simulink model "GuytonModel1972WithSubsystems_R2018_new"  (Simulink 9.1)
settings: Solver=ode23tb  StartTime=0.0  StopTime=inf  RelTol=1e-3  EnableMultiTasking=on
(part 1 of 3)
settings Model: LogicAnalyzerSignalOrdering=7aa3712b-a82d-49b1-ab79-c4b2009123cc,5a57f72a-0b0f-46f2-acdb-43125fd8ce03,a1eed3b7-a639-4f6e-9e66-41bbe214b6e5,0125497b-a83f-4e6f-858a-d937ae2b0d76,3e99b8dd-3e9c-45af-bc6c-72cad900a970,bdf28fdf-f6ee-494c-b426-144877683f61,daad667d-899e-428c-8c0c-82b3f4a58e16,7a1ec332-910d-4d5f-b535-061f2b58242f,8797777e-8256-4824-9350-18babea3f7fb,fa05effb-f5f0-4fb9-ae93-2c2ec5624b9e,8be5053f-f699-4e3b-912d-bda2fdf05311,7071d1a3-cbf6-4004-9a33-fb4c74e307a2,12eca2b8-30c7-4ca1-80c7-0d748863521c,1491594a-a680-41cf-9df3-666274efcfc0,a408ffc1-1556-4b3f-a007-6827623c9fa9,7caa9f0e-c1ef-45aa-8dd4-854c340c4311,cf932523-36ef-4960-9416-a49f3ce3abf4,5572dfed-c94c-4ac7-aa9a-9887f7f6c75f,825e1703-83b2-4867-8ebe-c975c17187a2,5d5b3bbb-1bff-46a6-a854-092626d3bdcf,2f97d808-bd79-4a93-951d-b9bb7f21fa84,3d0caab8-259e-423e-95e2-69965d32bdad,c121611d-42a5-4154-afc6-d4da5485fa77,4f2143c4-e6aa-439a-b86a-19df9d8919b1,a38d8fc3-90f2-40d7-afcb-4fa07d609ab0,d1aaf1a0-ab7d-4766-b05b-b674d56eddeb,9154d59b-3667-486d-a870-b223c724f572,4947b9e5-a051-4927-826b-f88022b127af,a5c37f39-2afb-4bf5-b5f4-deaa4e4f9e26,ab2d206b-5aa5-47ca-82a6-285e3435147c,a24f4fe4-8f8f-4ad5-bc1c-63b53242714e,d663d5fd-813e-4f3b-aebe-eaf2e7a06971,ca1ad65c-e5ef-44d1-86e8-ee4ec15310cd,a373b868-86f5-4960-8c53-9f982b71114b,b32a667a-ee1b-4402-8ab6-0e0293fa6f38,7e1f8eb4-0f51-4604-b00f-97ee570519ec,69dfedaa-aa11-44aa-8eef-81c2d931c5df,4045ec49-f8a0-442b-8ade-123442e10924,2a26ec00-979f-4a7b-8e9c-28a5bec13211,7373e241-3f2f-4e4f-91f7-b5466dda58a8,c9a36257-ac58-4413-a313-935ac06f1bc8  Creator=Jirka  LastModifiedBy=Jirka
settings DataIOCC: LimitDataPoints=on  MaxDataPoints=1000000  SaveFormat=Structure
settings OptimizationCC: ExpressionDepthLimit=2147483647  InitFltsAndDblsToZero=on
settings DebuggingCC: SaveWithParameterizedLinksMsg=none  SignalResolutionControl=TryResolveAllWithWarning  SolverPrmCheckMsg=warning  MultiTaskDSMMsg=warning  MultiTaskCondExecSysMsg=none  FcnCallInpInsideContextMsg=warning  StateNameClashWarn=warning
settings GRTTargetCC: TargetFcnLib=ansi_tfl_tmw.mat

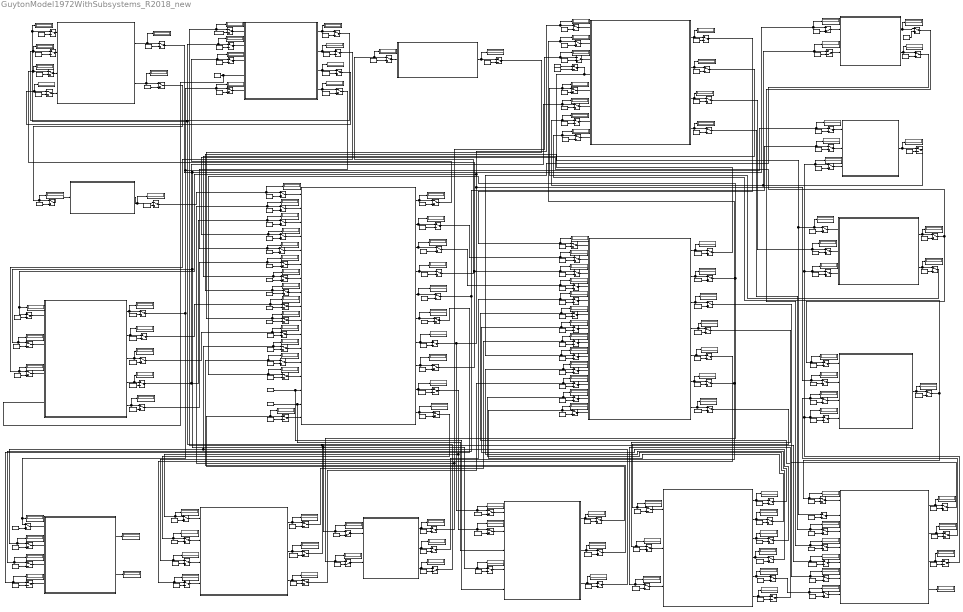
== system GuytonModel1972WithSubsystems_R2018_new ==
  note: PVS
  note: RVS
  note: BFN
  note: BFM
  note: PA
  note: PPA
  note: PRA
  note: PLA
  note: QLO
  note: VVE
  note: PC
  note: VV7
  note: VB
  note: VVR
  note: RBF
  note: AVE
  note: HPR
  note: HMD
  note: HPL
  note: ANM
  note: AMM
  note: AUM
  note: ARM
  note: VIM
  note: AUH
  note: HSR
  note: HSL
  note: AMM
  note: AOM
  note: P2O
  note: OVA
  note: AU
  note: EXC
  note: BFM
  note: HM
  note: VPF
  note: AUM
  note: PPC
  note: AM
  note: CNE
  note: AHM
  note: VIM
  note: REK
  note: PA
  note: AHM
  note: POT
  note: TVD
  note: STH
  note: AU
  note: CNA
  note: PRA
  note: RFN
  note: REK
  note: CNA
  note: CNE
  note: ANM
  note: RVS
  note: VUD
  note: BFN
  note: PVS
  note: VRC
  note: PIF
  note: PTC
  note: DFP
  note: TVD
  note: VTL
  note: PPD
  note: CPI
  note: DPL
  note: VB
  note: DPC
  note: PC
  note: VP
  note: CPP
  note: PPC
  note: VTC
  note: ANM
  note: PA
  note: CKE
  note: CNA
  note: AM
  note: DPC
  note: VTC
  note: VID
  note: CPI
  note: PTC
  note: DPL
  note: VTL
  note: VTS
  note: PIF
  note: PA
  note: PPA
  note: POT
  note: HPR
  note: HPL
  note: HMD
  note: POT
  note: VB
  note: HM
  note: VIM
  note: VRC
  note: PPA
  note: PLA
  note: CPP
  note: PPC
  note: VPF
  note: PPD
  note: DFP
  note: QLO
  note: HMD
  note: AU
  note: PRA
  note: AUM
  note: AVE
  note: AUH
  note: VVR
  note: AU
  note: POT
  note: EXC
  note: P2O
  note: PA
  note: POV
  note: ARM
  note: VID
  note: NOD
  note: STH
  note: VPF
  note: VP
  note: VTS
  note: CNA
  note: CKE
  note: VTW
  note: AM
  note: REK
  note: VUD
  note: RBF
  note: RFN
  note: NOD
  note: AHM
  note: NON-MUSCLE OXYGEN DELIVERY
  note: MUSCLE BLOOD FLOW CONTROL AND PO2
  note: VASCULAR STRESS RELAXATION
  note: KIDNEY DYNAMICS AND EXCRETION
  note: THIRST AND DRINKING
  note: ANTIDIURECTIC HORMONE CONTROL
  note: ALDOSTERONE CONTROL
  note: ANGIOTENSIN CONTROL
  note: ELECTROLYTES AND CELL WATER
  note: TISSUE FLUIDS, PRESSURES AND GEL
  note: HEART HYPERTROPHY OR DETERIORATION
  note: RED CELLS AND VISCOSITY
  note: PULMONARY DYNAMICS AND FLUIDS
  note: HEART RATE AND STROKE VOLUME
  note: AUTONOMIC CONTROL
  note: NON-MUSCLE LOCAL
      | BLOOD FLOW CONTROL
  note: CIRCULATORY DYNAMICS
  note: CAPILLARY MEMBRANE DYNAMICS
  AOM : Constant
  Aldosterone Control : Subsystem
      settings: MinAlgLoopOccurrences=on
      mask Display: disp('ALDOSTERONE CONTROL\n\nINTPUT:\nANM - angiotensin multiplier effect on vascular resistance,\n ratio to normal\nPA - aortic pressure [torr]\nCKE - extracellural potassium concentration \nCNA - extracellural sodium concentration \n\nOUTPUT:\nAM - aldosterone multiplier, ratio of normal effect\n')
  Angiotensin Control : Subsystem
      settings: MinAlgLoopOccurrences=on
      mask Display: disp('ANGIOTENSIN CONTROL\n\nINTPUTS:\nREK - percent of normal renal function\n [ratio to normal] \nRFN - renal blood flow if kidney is not damaged [l/min]\nCNA - extracellural sodium concentration \n\n\n OUTPUTS:\nANM - angiotensin multilier factor on vascular resistance\n [ratio to normal]\nCNE - sodium concentration abnormality causing third factor effect\n')
  Antidiurectic Hormone Control : Subsystem
      settings: MinAlgLoopOccurrences=on
      mask Display: disp('ANTIDIURECTIC HORMONE CONTROL\n\nINTPUT:\nAU - overall activity of autonomic system,\n ratio to normal \nPRA - right artial pressure \nCNA - extracellural sodium contrentration \n\nOUTPUT:\nAHM - antidiurectic hormone multiplifier,\n ratio of normal effect\n')
  Autonomic Control : Subsystem
      mask Display: disp('AUTONOMIC CONTROL \n\nINTPUTS:\nPA - systemic arterial pressure torr\nPOT - non-muscle cell PO2 [torr]\nP2O - muscle cell PO2  [torr]\nEXC - Effect of excercise on the metabolic usage of oxygen \nby the muscles [ratio to resting state]\nAUZ - overall sensitivity of autonomic control [ratio to normal]\n\nOUTPUTs:\nAU - overall activity af autonomic system\n[ratio to normal]\nAUH - autonomic multilier effect on the heart output\n[ratio to normal]\nVVR - basic volume of venous tree(maximum volume\n at zero pressure) [l]\nAUM - autonomic multipllier effect on arterial resistance \n[ratio to normal]\nAVE - autonomic multipllier effect on venous resistance\n[ratio to normal]\n')
  BFN : Constant  Value=2.8
  Capillary Membrane Dynamics : Subsystem
      mask Display: disp('CAPILLARY MEMBRANE DYNAMICS\n\nINTPUTS:\nPTC - colloid osmotic pressure of the tissue gel [torr]\nVTL - rate of return of fluid from the interstitium to the\nblood through the lymph [l/min]\nTVD - rate of intake of fluid by mounth or otherwise [l/min]\nRVS - venous resistance\nBFN - blood flow in non-muscle, non renal tissues\nPVS - average venous pressure\nVRC - volume of red blood cell\nVUD - rate of urinary output\nDFP - rate of increase in pulmonary free field\nPIF - intersticial fluid pressure\nPPD - rate od change of protein in pulmonary fluids\nCPI - concentration of protein in free intersticial fluid\nVP - plasma volume [l]\nDPL - rate of systemic lymphatic return of protela\n\nOUTPUTS:\nPC - systemic capillary pressure [torr]\nPPC - plasma colloid osmotic pressure [torr] \nVTC - toral rate of movement of fluid out of systemic capillaries[l/min]\nVB - blood volume\nCPP - plasma protein concentration\nDPC - rate of loss of plasma protein through systemic capillaries\n')
  Circulatory Dynamics : Subsystem
      settings: MinAlgLoopOccurrences=on
      mask Display: disp('CIRCULATORY DYNAMICS\n\nINTPUTS:\nARM - vasoconstrictor effect of all types of autoregulation\nVIM - blood viscosity (ratio to normal blood)\nAUM - sympathetic vasoconstrictor effect on arteries\nANM - angiotensin multiplier effect on vascular resistance, ratio to normal\nAMM - muscle vascular constriction caused by local tissue control, ratio to resting state\nAVE - sympathetic vasoconstrictor effect on veins\nRBF - renal blood flow [l/min]\nPC - capillary pressure  [torr]\nVVR - diminished vascular volume caused by sympathetic stimulation [l]\nVV7 - increased vascular volume caused by stress relaxation [l]\nAUH - autonomic stimulation of heart, ratio to normal\nHMD - cardiac depresant effect of hypoxia\nHPL - hypertrophy effect on left ventricle [ratio to normal]\nHPL - hypertrophy effect of left heart [ratio to normal]\nVB - blood volume [l]\nHSR - basic strenght or right ventricle [ratio to normal]\nHPR - hypertrophy effect of right heart [ratio to normal]\n\n\n  OUTPUTS:\nBFM - muscle blood flow [l/min]\nRVS - venous resistance [torr/l/min]\nPVS - average venous pressure  [torr]\nVVE - excess blood (stressed) volume in the systemic veins [l] \nPRA - right atrial pressure  [torr]\nQLO - output of left ventricle [l/min]\nPA - aortic pressure  [torr] \nBFN - blood flow in non-muscle, non-renal tissues [l/min]\nPRA - right atrial pressure  [torr]\nPLA - left atrial pressure  [torr]\n')
  Constant{1..2,4,95,106,189..190,196,198..201,205,209,213,216,234..235,241,245..249,254..257,259..260,274,280,283,285,295..297,299,304..306,308..309,322} (44 alike) : Constant
  Constant187 : Constant  Value=0.0125
  Constant188 : Constant  Value=40
  Constant192 : Constant  Value=0.3
  Constant{193,210,223,238,323} (5 alike) : Constant  Value=100
  Constant194 : Constant  Value=28
  Constant197 : Constant  Value=10
  Constant{202,221,231,236,253,268,271,275,281,286,302..303,320,325} (14 alike) : Constant  Value=0
  Constant{203,207,212,288} (4 alike) : Constant  Value=142
  Constant{204,226..227,239..240} (5 alike) : Constant  Value=8
  Constant{208,250,278..279} (4 alike) : Constant  Value=1.2
  Constant{211,229,237,258,267,287,290,315,324} (9 alike) : Constant  Value=5
  Constant215 : Constant  Value=0.1
  Constant217 : Constant  Value=0.0125
  Constant218 : Constant  Value=3
  Constant219 : Constant  Value=12
  Constant{220,270,291,313} (4 alike) : Constant  Value=0.002
  Constant{222,273,292,312} (4 alike) : Constant  Value=0.04
  Constant224 : Constant  Value=15
  Constant225 : Constant  Value=200
  Constant228 : Constant  Value=7.979
  Constant230 : Constant  Value=15
  Constant232 : Constant  Value=28
  Constant233 : Constant  Value=70
  Constant243 : Constant  Value=40
  Constant244 : Constant  Value=1.6
  Constant251 : Constant  Value=17
  Constant252 : Constant  Value=2.95
  Constant261 : Constant  Value=0.001
  Constant262 : Constant  Value=2.9
  Constant263 : Constant  Value=2.8
  Constant264 : Constant  Value=3.7
  Constant265 : Constant  Value=2
  Constant266 : Constant  Value=-6.3
  Constant269 : Constant  Value=0.001
  Constant272 : Constant  Value=20
  Constant276 : Constant  Value=0.001
  Constant277 : Constant  Value=0.1
  Constant284 : Constant  Value=10
  Constant289 : Constant  Value=12
  Constant293 : Constant  Value=-6.3
  Constant294 : Constant  Value=20
  Constant298 : Constant  Value=2
  Constant3 : Constant  Value=0.3
  Constant300 : Constant  Value=40
  Constant301 : Constant  Value=0.0125
  Constant307 : Constant  Value=2.95
  Constant310 : Constant  Value=3
  Constant311 : Constant  Value=70
  Constant314 : Constant  Value=17
  Constant316 : Constant  Value=28
  Constant317 : Constant  Value=3.7
  Constant318 : Constant  Value=2.9
  Constant319 : Constant  Value=0.3
  Constant321 : Constant  Value=2.8
  Constant326 : Constant  Value=15
  Display{1..143} (143 alike) : Display
  Electrolytes and Cell Water : Subsystem
      settings: MinAlgLoopOccurrences=on
      mask Display: disp('ELECTROLYTES AND CELL WATER\n\nINTPUTS:\nAM - aldosterone multiplier, ratio of normal effect\nREK - percent of normal renal function\n [ratio to normal] \nNOD - rate of excretion of sodium in the urine [mmol/min]\nSTH - salt appetite multiplier factor [ratio to normal]\nVTS - systemic interstitial fluid volume [l]\nVP - plasma volume [l]\nVPF - pulmonary interstitial fluid volume [l]\n\nOUTPUTS:\nVID - rate of fluid transfer between interstitial fluid and cells [l/min]\nCKE - extracellular potassium concentration [mmol/l]\nCNA - extracellular sodium concentration [mmol/l]\nVTW - total body water [l]\n')
  HM : Constant  Value=40
  Heart Hypertrophy or Deterioration : Subsystem
      settings: MinAlgLoopOccurrences=on
      mask Display: disp('HEART HYPERTROPHY OR DETERIORATION\n\nINTPUTS:\nPA - systemic arterial pressure [torr]\nPPA - pulmonary arterial pressure [torr]\nHSL - basic strenght or left ventricle [ratio to normal]\nPOT - Non muscle cells PO2 [troo]\nHSR - basic strenght or right ventricle [ratio to normal]\n\nOUTPUTS:\nHPR - hypertrophy effect of right heart [ratio to normal]\nHPL - hypertrophy effect of left heart [ratio to normal]\nHMD - cardiac depresant effect of hypoxia, shock\n')
  Heart Rate and Stroke Volume : Subsystem
      settings: MinAlgLoopOccurrences=on
      mask Display: disp('HEART RATE AND STROKE VOLUME\n\nINTPUTS:\nAUR - overall activity of autonomic system \n[ratio to normal] \nHMD - cardiac depresant effect of hypoxia, shock\nand other factors [ratio to normal] \nPRA - right atrial pressure [torr]\nQLO - output of left ventricle [l/min]\n\nOUTPUTS:\nSVO - stroke volume [l]\nHT - heart rate\n')
  Kidney  Dynamics and Excretion : Subsystem
      settings: MinAlgLoopOccurrences=on
      mask Display: disp('KIDNEY DYNAMICS AND EXCRETION\n\nINTPUTS:\nPA - aortic pressure [torr]\nPPC - plasma colloid osmotic pressure [torr] \nVIM - blood viscosity (ratio to normal blood \n[torr min/ll] \nREK - percent of normal renal function [ratio to normal] \nCNE - sodium concentration abnormability \ncausing third factor effect [mmol/l]\nAUM - sympathetic vasoconstrictor effect \non arteries [ratio of normal effect]\nAHM - antidiuretic hormone [ratio of normal effect]\nAM - aldosterone multiplier [ratio of normal effect] \n\n\n  OUTPUTS:\nVUD - rate of urinary output [l/min]\nRBF- renal blood flow [l/min]\nRFN - renal blood flow if kidney is not damaged [l/min]\nNOD - rate of renal excretion of sodium [mmol/min]\n\nAAR - afferent arteriolar resistance [torr min/l]\nEVR - postglomerular resistance [torr min/l]\nRR - renal resistance [torr min/l]\nGLP - glomerular pressure [torr]\nGFN - glomerular filtration rate of undamaged kidney [l/min]\nGFR - glomerular filtration rate [l/min]\n')
  Manual Switch{1..12,14..20,23..44,47..110,112..138,142..145} (136 alike) : ManualSwitch
  Manual Switch{13,21..22,45..46,111} (6 alike) : ManualSwitch  CurrentSetting=0
  Muscle Blood Flow Control And pO2 : Subsystem
      settings: MinAlgLoopOccurrences=on
      mask Display: disp('MUSCLE BLOOD FLOW CONTROL AND PO2\n\nINTPUTS:\nVPF - volume of free fluid in the pulmonary interstitium \nHM - hematocrit [%]\nBFM - blood flow in muscles \n [l/min]\nEXC - Effect of excercise on the metabolic usage \nof oxygen by the muscles [ratio to resting state]\nAU - overall activity of autonomic system\n  \nOUTPUTS:\nOVA - oxygen content of arterial blood \n[ml O2 STPD/l blood] \nP2O - muscle cell PO2  [torr]\nAOM - autonomic effect on tissue oxygenation \nAMM - muscle vascular constriction caused by logical tissue control\n[multiplifier, ratio to normal]\n\n')
  NON-MUSCLE OXYGEN DELIVERY : Subsystem
      mask Display: disp('NON-MUSCLE OXYGEN DELIVERY\n\nINTPUTS:\nHM-hematocrit [%]\nOVA-oxygen volume in aortic blood [ml O2/l blood]\nBFN-blood flow in non-muscle, non-renal tissues [l/min]\nAOM-autonomic effect on tissue oxygen utilization\n\nOUTPUTS:\nPOT-non-muscle cell PO2  [torr]\nPOV-non-muscle venous PO2 [torr]\n')
  "Non-Muscle Local Blood Flow Control " : Subsystem
      settings: MinAlgLoopOccurrences=on
      mask Display: disp('NON MUSCLE LOCAL BLOOD FLOW CONTROL\n\nINTPUT:\nPOT - non-muscle cells PO2 [torr] \n\nOUTPUT:\nARM - vasoconstrictor effect of local blood flow\n autoregulationin non-muscle tissues \n[ratio to normal]\n')
  OVA : Constant  Value=200
  POT : Constant  Value=8
  POV : Constant  Value=40
  Pulmonary Dynamics and Fluids : Subsystem
      mask Display: disp('PULMONARY DYNAMICS AND FLUIDS\n\nINTPUTS:\nPPA - pulmonary arterial pressure [torr]\nPLA - left atrial pressure [torr]\nPPC - plasma colloid osmotic pressure [torr]\nCPP - plasma protein concentration\n\nOUTPUTs:\nDFP - rate of change of free fluid in the lungs [l/min]\nVPF - volume of free fluid in the pulmonary interstitium [l/min]\nPPD - rate of loss of protein through the pulmonary capillary \nmembrane [g/min]\n')
  Red Cells And Viscosity : Subsystem
      settings: MinAlgLoopOccurrences=on
      mask Display: disp('RED CELLS AND VISCOSITY\n\nINTPUT:\nPOT - non-muscle cell PO2 [torr]\nVB - volume of blood [l]\n\nOUTPUT:\nVIM - blood viscosity [ratio to normal]\nHM - hematocrit [%]\nVRC - volume of red blood cells []\n')
  Thirst And Drinking : Subsystem
      settings: MinAlgLoopOccurrences=on
      mask Display: disp('THIRST AND DRINKING\n\nINTPUT:\nPOT - non muscle cells PO2 [torr] \nAHM - antidiurectical hormone effect to non renal\n vascular resistance, multiplifier \n(ratio to normal effect)\nOUTPUT:\nSTH - salt appetite multiplifier factor\n [ratio to normal]  \nTVD - rate of intake of fluid by mouth \n or otherwise [l/min]\n')
  "Tissue Fluids, Pressures and Gel" : Subsystem
      mask Display: disp('TISSUE FLUIDS, PRESSURES AND GEL\n\nINTPUTS:\nVTC - rate of fluid transfer across systemic intersticial fluid\nDPC -rate of influx protein into the interstitial fluid from plasma [g/min]\nVID - rate of fluid transfer between interstitial fluid and cells\n\nOUTPUTs:\nPTC - total colloid osmotic pressure of the tissue gel]\nVTL - lymph flow rate [l/min]\nDPL - rate of return of protein to the circulatin by way of the lymph [g/min]\nCPI - concentration pf protein in the interstitium [g/l]\nVTS - total interstitial fluid volume [l]\n')
  Vascular Stress Relaxation : Subsystem
      settings: MinAlgLoopOccurrences=on
      mask Display: disp('VASCULAR STRESS RELAXATION\n\nINTPUT:\nVVE - VVE - excess blood (stressed) volume in the veins [l] \n \n\nOUTPUT:\nVV7 - increased vascular volume caused by stress relaxation [l] \n')
  wires:
  Circulatory Dynamics/3(PVS) -> Manual Switch129/1, Display2/1
  Constant317/1 -> Manual Switch129/2
  Circulatory Dynamics/2(RVS) -> Manual Switch130/1, Display1/1
  Constant318/1 -> Manual Switch130/2
  Constant321/1 -> Manual Switch133/2
  Circulatory Dynamics/1(BFM) -> Manual Switch134/1, Display35/1
  Constant322/1 -> Manual Switch134/2
  Circulatory Dynamics/7(PA) -> Manual Switch135/1, Display6/1
  Constant323/1 -> Manual Switch135/2
  Circulatory Dynamics/8(BFN) -> Manual Switch133/1, Display7/1
  Constant326/1 -> Manual Switch138/2
  Circulatory Dynamics/5(PRA) -> Manual Switch132/1, Display4/1
  Constant320/1 -> Manual Switch132/2
  Circulatory Dynamics/9(PPA) -> Manual Switch138/1, Display8/1
  Circulatory Dynamics/10(PLA) -> Manual Switch137/1, Display9/1
  Constant325/1 -> Manual Switch137/2
  Circulatory Dynamics/6(QLO) -> Manual Switch136/1, Display5/1
  Constant324/1 -> Manual Switch136/2
  Circulatory Dynamics/4(VVE) -> Manual Switch131/1, Display3/1
  Constant319/1 -> Manual Switch131/2
  Manual Switch68/1 -> Circulatory Dynamics/8(PC)
  Constant251/1 -> Manual Switch68/2
  Manual Switch70/1 -> Circulatory Dynamics/10(VV7)
  Constant253/1 -> Manual Switch70/2
  Manual Switch75/1 -> Circulatory Dynamics/14(VB)
  Constant258/1 -> Manual Switch75/2
  Manual Switch69/1 -> Circulatory Dynamics/9(VVR)
  Constant252/1 -> Manual Switch69/2
  Manual Switch67/1 -> Circulatory Dynamics/7(RBF)
  Constant250/1 -> Manual Switch67/2
  Manual Switch66/1 -> Circulatory Dynamics/6(AVE)
  Constant249/1 -> Manual Switch66/2
  Manual Switch77/1 -> Circulatory Dynamics/17(HPR)
  Constant260/1 -> Manual Switch77/2
  Manual Switch72/1 -> Circulatory Dynamics/12(HMD)
  Constant255/1 -> Manual Switch72/2
  Manual Switch73/1 -> Circulatory Dynamics/13(HPL)
  Constant256/1 -> Manual Switch73/2
  Manual Switch64/1 -> Circulatory Dynamics/4(ANM)
  Constant247/1 -> Manual Switch64/2
  Manual Switch65/1 -> Circulatory Dynamics/5(AMM)
  Constant248/1 -> Manual Switch65/2
  Manual Switch63/1 -> Circulatory Dynamics/3(AUM)
  Constant246/1 -> Manual Switch63/2
  Manual Switch61/1 -> Circulatory Dynamics/1(ARM)
  Constant244/1 -> Manual Switch61/2
  Manual Switch62/1 -> Circulatory Dynamics/2(VIM)
  Constant245/1 -> Manual Switch62/2
  Manual Switch71/1 -> Circulatory Dynamics/11(AUH)
  Constant254/1 -> Manual Switch71/2
  Constant259/1 -> Circulatory Dynamics/15(HSR), Heart Hypertrophy or Deterioration/5(HSR)
  Constant257/1 -> Circulatory Dynamics/16(HSL), Heart Hypertrophy or Deterioration/3(HSL)
  Manual Switch142/1 -> NON-MUSCLE OXYGEN DELIVERY/1(HM)
  Manual Switch143/1 -> NON-MUSCLE OXYGEN DELIVERY/2(OVA)
  Manual Switch144/1 -> NON-MUSCLE OXYGEN DELIVERY/3(BFN)
  Manual Switch145/1 -> NON-MUSCLE OXYGEN DELIVERY/4(AOM)
  NON-MUSCLE OXYGEN DELIVERY/1(POT) -> Display11/1, Manual Switch1/1
  POT/1 -> Manual Switch1/2
  NON-MUSCLE OXYGEN DELIVERY/2(POV) -> Display10/1, Manual Switch2/1
  POV/1 -> Manual Switch2/2
  HM/1 -> Manual Switch142/2
  OVA/1 -> Manual Switch143/2
  BFN/1 -> Manual Switch144/2
  AOM/1 -> Manual Switch145/2
  Manual Switch4/1 -> Muscle Blood Flow Control And pO2/1(VPF)
  Manual Switch5/1 -> Muscle Blood Flow Control And pO2/2(HM)
  Manual Switch6/1 -> Muscle Blood Flow Control And pO2/3(BFM)
  Manual Switch8/1 -> Muscle Blood Flow Control And pO2/5(AU)
  Muscle Blood Flow Control And pO2/4(AMM) -> Manual Switch42/1, Display19/1
  Constant241/1 -> Manual Switch42/2
  Muscle Blood Flow Control And pO2/3(AOM) -> Manual Switch43/1, Display17/1
  Constant274/1 -> Manual Switch43/2
  Muscle Blood Flow Control And pO2/2(P2O) -> Manual Switch31/1, Display15/1
  Constant226/1 -> Manual Switch31/2
  Constant225/1 -> Manual Switch23/2
  Muscle Blood Flow Control And pO2/1(OVA) -> Manual Switch23/1, Display16/1
  Constant189/1 -> Manual Switch6/2
  Constant188/1 -> Manual Switch5/2
  Constant187/1 -> Manual Switch4/2
  Constant1/1 -> Manual Switch8/2
  Constant192/1 -> Manual Switch9/2
  Manual Switch9/1 -> Vascular Stress Relaxation/1(VVE)
  Vascular Stress Relaxation/1(VV7) -> Manual Switch58/1, Display21/1
  Constant275/1 -> Manual Switch58/2
  Constant198/1 -> Manual Switch15/2
  Manual Switch15/1 -> Kidney  Dynamics and Excretion/6(AUM)
  Manual Switch11/1 -> Kidney  Dynamics and Excretion/2(PPC)
  Constant194/1 -> Manual Switch11/2
  Manual Switch17/1 -> Kidney  Dynamics and Excretion/8(AM)
  Constant200/1 -> Manual Switch17/2
  Manual Switch14/1 -> Kidney  Dynamics and Excretion/5(CNE)
  Constant197/1 -> Manual Switch14/2
  Manual Switch16/1 -> Kidney  Dynamics and Excretion/7(AHM)
  Constant199/1 -> Manual Switch16/2
  Manual Switch13/1 -> Kidney  Dynamics and Excretion/3(VIM)
  Constant196/1 -> Manual Switch13/2
  Manual Switch10/1 -> Kidney  Dynamics and Excretion/1(PA)
  Constant193/1 -> Manual Switch10/2
  Kidney  Dynamics and Excretion/3(RFN) -> Manual Switch74/1, Display30/1
  Constant279/1 -> Manual Switch74/2
  Kidney  Dynamics and Excretion/4(NOD) -> Manual Switch91/1, Display31/1
  Constant277/1 -> Manual Switch91/2
  Kidney  Dynamics and Excretion/1(VUD) -> Manual Switch76/1, Display32/1
  Constant276/1 -> Manual Switch76/2
  Kidney  Dynamics and Excretion/2(RBF) -> Manual Switch59/1, Display23/1
  Constant278/1 -> Manual Switch59/2
  Manual Switch21/1 -> Thirst And Drinking/1(POT)
  Constant204/1 -> Manual Switch21/2
  Manual Switch22/1 -> Thirst And Drinking/2(AHM)
  Thirst And Drinking/2(TVD) -> Manual Switch93/1, Display34/1
  Thirst And Drinking/1(STH) -> Manual Switch92/1, Display37/1
  Constant205/1 -> Manual Switch22/2
  Manual Switch20/1 -> Antidiurectic Hormone Control/3(CNA)
  Constant203/1 -> Manual Switch20/2
  Constant201/1 -> Manual Switch18/2
  Manual Switch18/1 -> Antidiurectic Hormone Control/1(AU)
  Manual Switch19/1 -> Antidiurectic Hormone Control/2(PRA)
  Constant202/1 -> Manual Switch19/2
  Antidiurectic Hormone Control/1(AHM) -> Manual Switch94/1, Display39/1
  Constant2/1 -> Manual Switch94/2
  Manual Switch25/1 -> Angiotensin Control/2(RFN)
  Constant208/1 -> Manual Switch25/2
  Manual Switch24/1 -> Angiotensin Control/3(CNA)
  Constant207/1 -> Manual Switch24/2
  Angiotensin Control/2(CNE) -> Manual Switch96/1, Display43/1
  Constant284/1 -> Manual Switch96/2
  Angiotensin Control/1(ANM) -> Manual Switch95/1, Display45/1
  Constant283/1 -> Manual Switch95/2
  Manual Switch79/1 -> Capillary Membrane Dynamics/2(RVS)
  Constant262/1 -> Manual Switch79/2
  Manual Switch78/1 -> Capillary Membrane Dynamics/1(VUD)
  Constant261/1 -> Manual Switch78/2
  Constant263/1 -> Manual Switch80/2
  Manual Switch80/1 -> Capillary Membrane Dynamics/3(BFN)
  Manual Switch81/1 -> Capillary Membrane Dynamics/4(PVS)
  Constant264/1 -> Manual Switch81/2
  Constant265/1 -> Manual Switch82/2
  Manual Switch82/1 -> Capillary Membrane Dynamics/5(VRC)
  Constant266/1 -> Manual Switch83/2
  Manual Switch83/1 -> Capillary Membrane Dynamics/6(PIF)
  Constant267/1 -> Manual Switch84/2
  Manual Switch84/1 -> Capillary Membrane Dynamics/7(PTC)
  Constant268/1 -> Manual Switch85/2
  Manual Switch85/1 -> Capillary Membrane Dynamics/8(DFP)
  Constant269/1 -> Manual Switch86/2
  Manual Switch86/1 -> Capillary Membrane Dynamics/9(TVD)
  Constant270/1 -> Manual Switch87/2
  Manual Switch87/1 -> Capillary Membrane Dynamics/10(VTL)
  Constant271/1 -> Manual Switch88/2
  Manual Switch88/1 -> Capillary Membrane Dynamics/11(PPD)
  Manual Switch89/1 -> Capillary Membrane Dynamics/12(CPI)
  Constant272/1 -> Manual Switch89/2
  Manual Switch90/1 -> Capillary Membrane Dynamics/13(DPL)
  Constant273/1 -> Manual Switch90/2
  Capillary Membrane Dynamics/2(VB) -> Manual Switch126/1, Display50/1
  Constant315/1 -> Manual Switch126/2
  Constant312/1 -> Manual Switch127/2
  Capillary Membrane Dynamics/4(DPC) -> Manual Switch127/1, Display51/1
  Capillary Membrane Dynamics/1(PC) -> Manual Switch125/1, Display52/1
  Constant314/1 -> Manual Switch125/2
  Capillary Membrane Dynamics/3(VP) -> Manual Switch122/1, Display53/1
  Constant310/1 -> Manual Switch122/2
  Capillary Membrane Dynamics/5(CPP) -> Manual Switch128/1, Display54/1
  Constant311/1 -> Manual Switch128/2
  Capillary Membrane Dynamics/6(PPC) -> Manual Switch123/1, Display55/1
  Constant316/1 -> Manual Switch123/2
  Capillary Membrane Dynamics/7(VTC) -> Manual Switch124/1, Display56/1
  Constant313/1 -> Manual Switch124/2
  Manual Switch26/1 -> Aldosterone Control/1(ANM)
  Constant209/1 -> Manual Switch26/2
  Manual Switch27/1 -> Aldosterone Control/2(PA)
  Constant210/1 -> Manual Switch27/2
  Manual Switch28/1 -> Aldosterone Control/3(CKE)
  Constant211/1 -> Manual Switch28/2
  Manual Switch29/1 -> Aldosterone Control/4(CNA)
  Constant212/1 -> Manual Switch29/2
  Aldosterone Control/1(AM) -> Manual Switch97/1, Display74/1
  Constant285/1 -> Manual Switch97/2
  Manual Switch39/1 -> "Tissue Fluids, Pressures and Gel"/2(DPC)
  Constant222/1 -> Manual Switch39/2
  Manual Switch37/1 -> "Tissue Fluids, Pressures and Gel"/1(VTC)
  Constant220/1 -> Manual Switch37/2
  Manual Switch38/1 -> "Tissue Fluids, Pressures and Gel"/3(VID)
  Constant221/1 -> Manual Switch38/2
  "Tissue Fluids, Pressures and Gel"/4(CPI) -> Manual Switch105/1, Display87/1
  Constant294/1 -> Manual Switch105/2
  "Tissue Fluids, Pressures and Gel"/3(PTC) -> Manual Switch106/1, Display89/1
  Constant290/1 -> Manual Switch106/2
  "Tissue Fluids, Pressures and Gel"/2(DPL) -> Manual Switch104/1, Display90/1
  Constant292/1 -> Manual Switch104/2
  "Tissue Fluids, Pressures and Gel"/1(VTL) -> Manual Switch103/1, Display91/1
  Constant291/1 -> Manual Switch103/2
  "Tissue Fluids, Pressures and Gel"/5(VTS) -> Manual Switch101/1, Display92/1
  Constant289/1 -> Manual Switch101/2
  "Tissue Fluids, Pressures and Gel"/6(PIF) -> Manual Switch102/1, Display93/1
  Constant293/1 -> Manual Switch102/2
  Constant223/1 -> Manual Switch40/2
  Manual Switch40/1 -> Heart Hypertrophy or Deterioration/1(PA)
  Constant224/1 -> Manual Switch41/2
  Manual Switch41/1 -> Heart Hypertrophy or Deterioration/2(PPA)
  Manual Switch44/1 -> Heart Hypertrophy or Deterioration/4(POT)
  Constant227/1 -> Manual Switch44/2
  Heart Hypertrophy or Deterioration/1(HPR) -> Manual Switch108/1, Display99/1
  Constant296/1 -> Manual Switch108/2
  Heart Hypertrophy or Deterioration/2(HPL) -> Manual Switch109/1, Display100/1
  Constant297/1 -> Manual Switch109/2
  Heart Hypertrophy or Deterioration/3(HMD) -> Manual Switch107/1, Display101/1
  Constant295/1 -> Manual Switch107/2
  Manual Switch45/1 -> Red Cells And Viscosity/1(POT)
  Constant228/1 -> Manual Switch45/2
  Manual Switch46/1 -> Red Cells And Viscosity/2(VB)
  Constant229/1 -> Manual Switch46/2
  Red Cells And Viscosity/3(HM) -> Manual Switch111/1, Display105/1
  Constant300/1 -> Manual Switch111/2
  Red Cells And Viscosity/1(VIM) -> Manual Switch112/1, Display103/1
  Constant299/1 -> Manual Switch112/2
  Red Cells And Viscosity/2(VRC) -> Manual Switch110/1, Display104/1
  Constant298/1 -> Manual Switch110/2
  Manual Switch47/1 -> Pulmonary Dynamics and Fluids/1(PPA)
  Constant230/1 -> Manual Switch47/2
  Manual Switch48/1 -> Pulmonary Dynamics and Fluids/2(PLA)
  Constant231/1 -> Manual Switch48/2
  Constant233/1 -> Manual Switch50/2
  Manual Switch50/1 -> Pulmonary Dynamics and Fluids/4(CPP)
  Manual Switch49/1 -> Pulmonary Dynamics and Fluids/3(PPC)
  Constant232/1 -> Manual Switch49/2
  Pulmonary Dynamics and Fluids/2(VPF) -> Manual Switch114/1, Display112/1
  Constant301/1 -> Manual Switch114/2
  Pulmonary Dynamics and Fluids/3(PPD) -> Manual Switch113/1, Display113/1
  Constant303/1 -> Manual Switch113/2
  Pulmonary Dynamics and Fluids/1(DFP) -> Manual Switch115/1, Display110/1
  Constant302/1 -> Manual Switch115/2
  Constant237/1 -> Manual Switch54/2
  Manual Switch54/1 -> Heart Rate and Stroke Volume/4(QLO)
  Heart Rate and Stroke Volume/1(SVO) -> Display114/1
  Constant235/1 -> Manual Switch52/2
  Manual Switch52/1 -> Heart Rate and Stroke Volume/2(HMD)
  Manual Switch51/1 -> Heart Rate and Stroke Volume/1(AU)
  Constant234/1 -> Manual Switch51/2
  Manual Switch53/1 -> Heart Rate and Stroke Volume/3(PRA)
  Constant236/1 -> Manual Switch53/2
  Autonomic Control/4(AUM) -> Manual Switch117/1, Display117/1
  Constant305/1 -> Manual Switch117/2
  Constant304/1 -> Manual Switch116/2
  Autonomic Control/5(AVE) -> Manual Switch116/1, Display118/1
  Autonomic Control/3(AUH) -> Manual Switch118/1, Display116/1
  Constant306/1 -> Manual Switch118/2
  Autonomic Control/2(VVR) -> Manual Switch119/1, Display115/1
  Constant307/1 -> Manual Switch119/2
  Autonomic Control/1(AU) -> Manual Switch120/1, Display119/1
  Constant308/1 -> Manual Switch120/2
  Manual Switch56/1 -> Autonomic Control/2(POT)
  Constant239/1 -> Manual Switch56/2
  Constant190/1 -> Autonomic Control/4(EXC), Muscle Blood Flow Control And pO2/4(EXC)
  Manual Switch57/1 -> Autonomic Control/3(P2O)
  Constant240/1 -> Manual Switch57/2
  Manual Switch55/1 -> Autonomic Control/1(PA)
  Constant238/1 -> Manual Switch55/2
  Manual Switch60/1 -> "Non-Muscle Local Blood Flow Control "/1(POV)
  Constant243/1 -> Manual Switch60/2
  "Non-Muscle Local Blood Flow Control "/1(ARM) -> Manual Switch121/1, Display120/1
  Constant309/1 -> Manual Switch121/2
  Electrolytes and Cell Water/1(VID) -> Manual Switch98/1, Display77/1
  Constant286/1 -> Manual Switch98/2
  Constant215/1 -> Manual Switch32/2
  Manual Switch32/1 -> Electrolytes and Cell Water/3(NOD)
  Manual Switch33/1 -> Electrolytes and Cell Water/4(STH)
  Constant216/1 -> Manual Switch33/2
  Manual Switch34/1 -> Electrolytes and Cell Water/5(VPF)
  Constant217/1 -> Manual Switch34/2
  Manual Switch35/1 -> Electrolytes and Cell Water/6(VP)
  Constant218/1 -> Manual Switch35/2
  Manual Switch36/1 -> Electrolytes and Cell Water/7(VTS)
  Constant219/1 -> Manual Switch36/2
  Electrolytes and Cell Water/3(CNA) -> Manual Switch100/1, Display81/1
  Constant288/1 -> Manual Switch100/2
  Electrolytes and Cell Water/2(CKE) -> Manual Switch99/1, Display82/1
  Constant287/1 -> Manual Switch99/2
  Electrolytes and Cell Water/4(VTW) -> Display83/1
  Manual Switch30/1 -> Electrolytes and Cell Water/1(AM)
  Constant213/1 -> Manual Switch30/2
  Manual Switch111/1 -> Manual Switch142/1, Display64/1, Manual Switch5/1, Display12/1
  Manual Switch23/1 -> Manual Switch143/1, Display63/1
  Manual Switch133/1 -> Manual Switch144/1, Display62/1, Manual Switch80/1, Display57/1
  Manual Switch43/1 -> Manual Switch145/1, Display61/1
  Manual Switch114/1 -> Manual Switch4/1, Display18/1, Manual Switch34/1, Display78/1
  Manual Switch115/1 -> Manual Switch85/1, Display67/1
  Manual Switch134/1 -> Manual Switch6/1, Display13/1
  Manual Switch120/1 -> Manual Switch8/1, Display14/1, Manual Switch18/1, Display38/1, Manual Switch51/1, Display138/1
  Manual Switch131/1 -> Display20/1, Manual Switch9/1
  Manual Switch135/1 -> Manual Switch27/1, Display70/1, Manual Switch10/1, Display28/1, Manual Switch55/1, Display135/1, Manual Switch40/1, Display95/1
  Manual Switch123/1 -> Manual Switch11/1, Display22/1, Manual Switch49/1, Display108/1
  Manual Switch112/1 -> Manual Switch13/1, Display27/1, Manual Switch62/1, Display98/1
  Manual Switch96/1 -> Manual Switch14/1, Display25/1
  Manual Switch117/1 -> Manual Switch15/1, Display29/1, Manual Switch63/1, Display122/1
  Manual Switch94/1 -> Manual Switch16/1, Display26/1, Manual Switch22/1, Display33/1
  Manual Switch97/1 -> Manual Switch17/1, Display24/1, Manual Switch30/1, Display84/1
  Manual Switch1/1 -> Manual Switch21/1, Display36/1, Manual Switch45/1, Display106/1, Manual Switch44/1, Display96/1, Manual Switch56/1, Display136/1
  Manual Switch132/1 -> Manual Switch19/1, Display41/1, Manual Switch53/1, Display140/1
  Manual Switch100/1 -> Manual Switch29/1, Display73/1, Manual Switch24/1, Display42/1, Display40/1, Manual Switch20/1
  Manual Switch74/1 -> Manual Switch25/1, Display44/1
  Manual Switch95/1 -> Manual Switch64/1, Display123/1, Manual Switch26/1, Display72/1
  Manual Switch99/1 -> Manual Switch28/1, Display71/1
  Manual Switch91/1 -> Manual Switch32/1, Display75/1
  Manual Switch92/1 -> Manual Switch33/1, Display76/1
  Manual Switch122/1 -> Manual Switch35/1, Display79/1
  Manual Switch101/1 -> Manual Switch36/1, Display80/1
  Manual Switch124/1 -> Manual Switch37/1, Display85/1
  Manual Switch127/1 -> Manual Switch39/1, Display88/1
  Manual Switch98/1 -> Manual Switch38/1, Display86/1
  Manual Switch138/1 -> Manual Switch41/1, Display94/1, Manual Switch47/1, Display111/1
  Manual Switch126/1 -> Manual Switch46/1, Display102/1, Manual Switch75/1, Display133/1
  Manual Switch2/1 -> Manual Switch60/1, Display121/1
  Manual Switch121/1 -> Manual Switch61/1, Display97/1
  Manual Switch31/1 -> Manual Switch57/1, Display137/1
  Manual Switch107/1 -> Manual Switch52/1, Display139/1, Manual Switch72/1, Display131/1
  Manual Switch136/1 -> Manual Switch54/1, Display141/1
  Manual Switch137/1 -> Manual Switch48/1, Display107/1
  Manual Switch128/1 -> Manual Switch50/1, Display109/1
  Manual Switch42/1 -> Manual Switch65/1, Display124/1
  Manual Switch116/1 -> Manual Switch66/1, Display125/1
  Manual Switch59/1 -> Manual Switch67/1, Display126/1
  Manual Switch125/1 -> Manual Switch68/1, Display127/1
  Manual Switch119/1 -> Manual Switch69/1, Display128/1
  Manual Switch58/1 -> Manual Switch70/1, Display129/1
  Manual Switch118/1 -> Manual Switch71/1, Display130/1
  Manual Switch109/1 -> Manual Switch73/1, Display132/1
  Manual Switch108/1 -> Manual Switch77/1, Display134/1
  Manual Switch76/1 -> Manual Switch78/1, Display46/1
  Manual Switch130/1 -> Manual Switch79/1, Display59/1
  Manual Switch129/1 -> Manual Switch81/1, Display58/1
  Manual Switch110/1 -> Manual Switch82/1, Display60/1
  Manual Switch102/1 -> Manual Switch83/1, Display65/1
  Manual Switch106/1 -> Manual Switch84/1, Display66/1
  Manual Switch93/1 -> Manual Switch86/1, Display68/1
  Manual Switch103/1 -> Manual Switch87/1, Display69/1
  Manual Switch113/1 -> Manual Switch88/1, Display47/1
  Manual Switch105/1 -> Manual Switch89/1, Display48/1
  Manual Switch104/1 -> Manual Switch90/1, Display49/1
  Heart Rate and Stroke Volume/2(HR) -> Display142/1
  Manual Switch3/1 -> Angiotensin Control/1(REK)
  Constant95/1 -> Manual Switch3/2
  Manual Switch7/1 -> Electrolytes and Cell Water/2(REK)
  Constant106/1 -> Manual Switch7/2
  Manual Switch12/1 -> Kidney  Dynamics and Excretion/4(REK), Manual Switch7/1, Manual Switch3/1, Display143/1
  Constant3/1 -> Manual Switch12/2
  Constant281/1 -> Manual Switch93/2
  Constant280/1 -> Manual Switch92/2
  Constant4/1 -> Manual Switch12/1

== system GuytonModel1972WithSubsystems_R2018_new/Aldosterone Control ==
  note: 173
  note: AM3
  note: AM2
  note: AMC
  note: KN1
  note: 168
  note: AMP
  note: 171
  note: 172
  note: 174
  note: AM1
  note: AMR
  note: AM5
  note: 166
  note: 165
  note: ALDOSTERONE CONTROL
  note: AMT
  note: 169
  note: 167
  note: 170
  note: 164
  ANM : Inport
  PA : Inport  Port=2
  CKE : Inport  Port=3
  CNA : Inport  Port=4
  AMP = f(PA)1 : Subsystem
      mask Display:
      | plot([ 0    10    20    30    40    50    60    70    80    90   100   110   120   130   140   150   160   170   180   190   200], [4.0000    3.6505    3.3040    2.9635    2.6320    2.3125    2.0080    1.7215    1.4560    1.2145    1.0000    0.8145    0.6560    0.5215    0.4080    0.3125    0.2320    0.1635    0.1040    0.0505    0.0000])
      | 
      | text(-20,2,'')
      | text(230,2,'')
      | text(100,4.2,'')
      | text(100,-0.4,'')
      | 
      | text(-16,0,'0')
      | text(0,-0.2,'0')
      | text(-16,4,'4')
      | text(190,-0.2,'200')
  Constant1 : Constant  Value=9
  Constant2 : Constant  Value=60
  Constant3 : Constant  Value=-0.017
  Constant4 : Constant  Value=19.8
  Constant5 : Constant  Value=20.039
  Constant6 : Constant  Value=0.00352
  KE 1 : Integrator  InitialConditionSource=external  InitialCondition=74.7024
  Math Function1 : Math  Operator=10^u  SaturateOnIntegerOverflow=on
  Product1 : Product  Inputs=/*  SaturateOnIntegerOverflow=on  RndMeth=Zero  InputSameDT=on  OutDataTypeStr=Inherit: Same as first input
  Product2 : Product  Inputs=3  SaturateOnIntegerOverflow=on  RndMeth=Zero  InputSameDT=on  OutDataTypeStr=Inherit: Same as first input
  Product3 : Product  SaturateOnIntegerOverflow=on  RndMeth=Zero  InputSameDT=on  OutDataTypeStr=Inherit: Same as first input
  Product4 : Product  Inputs=/*/  SaturateOnIntegerOverflow=on  RndMeth=Zero  InputSameDT=on  OutDataTypeStr=Inherit: Same as first input
  Product5 : Product  SaturateOnIntegerOverflow=on  RndMeth=Zero  InputSameDT=on  OutDataTypeStr=Inherit: Same as first input
  Sum1 : Sum  Inputs=|+-  SaturateOnIntegerOverflow=on  InputSameDT=on  OutDataTypeStr=Inherit: Same as first input
  Sum2 : Sum  Inputs=+|-  SaturateOnIntegerOverflow=on  InputSameDT=on  OutDataTypeStr=Inherit: Same as first input
  Sum3 : Sum  Inputs=+-|  SaturateOnIntegerOverflow=on  InputSameDT=on  OutDataTypeStr=Inherit: Same as first input
  Z1 : Constant
  lower limit 1 : Saturate  UpperLimit=inf  LowerLimit=0  LinearizeAsGain=off
  AM : Outport
  wires:
  KE 1/1 -> Sum2/2, Product3/2
  PA/1 -> AMP = f(PA)1/1(PA)
  Math Function1/1 -> Product5/2
  Constant1/1 -> Sum1/2
  Product5/1 -> Sum3/2
  Constant6/1 -> Product4/1
  Sum1/1 -> lower limit 1/1
  Constant3/1 -> Product3/1
  Constant4/1 -> Product5/1
  AMP = f(PA)1/1(AMP) -> Product2/2
  Product1/1 -> KE 1/1
  Constant2/1 -> Product1/1
  Product2/1 -> Sum2/1
  Sum2/1 -> Product1/2
  Product3/1 -> Math Function1/1
  Product4/1 -> Sum1/1
  Z1/1 -> KE 1/2
  lower limit 1/1 -> Product2/3
  Constant5/1 -> Sum3/1
  CNA/1 -> Product4/3
  CKE/1 -> Product4/2
  ANM/1 -> Product2/1
  Sum3/1 -> AM/1

== system GuytonModel1972WithSubsystems_R2018_new/Angiotensin Control ==
  note: 159
  note: 154
  note: 160
  note: 153a
  note: ANT
  note: 153b
  note: ANC
  note: ANGIOTENSIN CONTROL
  note: AN1
  note: AN2
  note: 155
  note: AN3
  note: 163
  note: AN5
  note: 156
  note: 161
  note: 162
  note: 157
  note: 158
  REK : Inport
  RFN : Inport  Port=2
  CNA : Inport  Port=3
  (1.2/RFN)^1 : Fcn  Expr=(1.2/u)^3
  Constant1 : Constant  Value=152
  Constant2 : Constant  Value=0.1
  Constant3 : Constant  Value=15
  Constant4 : Constant  Value=0.042
  Constant5 : Constant  Value=3.3
  Constant6 : Constant  Value=4.0
  Integrator1 : Integrator  InitialConditionSource=external
  Math Function1 : Math  Operator=10^u  SaturateOnIntegerOverflow=on
  Product{1..3,6} (4 alike) : Product  SaturateOnIntegerOverflow=on  RndMeth=Zero  InputSameDT=on  OutDataTypeStr=Inherit: Same as first input
  Product4 : Product  Inputs=*/  SaturateOnIntegerOverflow=on  RndMeth=Zero  InputSameDT=on  OutDataTypeStr=Inherit: Same as first input
  Product5 : Product  Inputs=*/  SaturateOnIntegerOverflow=on  RndMeth=Zero  InputSameDT=on  OutDataTypeStr=Inherit: Same as first input
  Sum1 : Sum  Inputs=|-+  SaturateOnIntegerOverflow=on  InputSameDT=on  OutDataTypeStr=Inherit: Same as first input
  Sum2 : Sum  Inputs=-+|  SaturateOnIntegerOverflow=on  InputSameDT=on  OutDataTypeStr=Inherit: Same as first input
  Sum3 : Sum  Inputs=|-+  SaturateOnIntegerOverflow=on  InputSameDT=on  OutDataTypeStr=Inherit: Same as first input
  Xo1 : Constant  VectorParams1D=off
  lower limit 0.7 : Saturate  UpperLimit=inf  LowerLimit=0.7  LinearizeAsGain=off
  ANM : Outport
  CNE : Outport  Port=2
  wires:
  Sum1/1 -> CNE/1, Product2/1
  Product5/1 -> Sum3/1
  Product3/1 -> Math Function1/1
  Product4/1 -> Integrator1/1
  Product6/1 -> Product1/1  "ANP"
  Constant6/1 -> Sum3/2
  RFN/1 -> (1.2/RFN)^1/1
  Product1/1 -> Sum2/2
  Constant3/1 -> Product4/2  "ANT"
  Sum3/1 -> lower limit 0.7/1
  Constant5/1 -> Product5/1
  Math Function1/1 -> Product5/2
  Constant1/1 -> Sum1/2
  Sum2/1 -> Product4/1
  Product2/1 -> Product1/2  "ANN"
  (1.2/RFN)^1/1 -> Product6/2
  Constant2/1 -> Product2/2
  Constant4/1 -> Product3/1
  Xo1/1 -> Integrator1/2
  Integrator1/1 -> Sum2/1, Product3/2  "ANC"
  REK/1 -> Product6/1
  CNA/1 -> Sum1/1
  lower limit 0.7/1 -> ANM/1

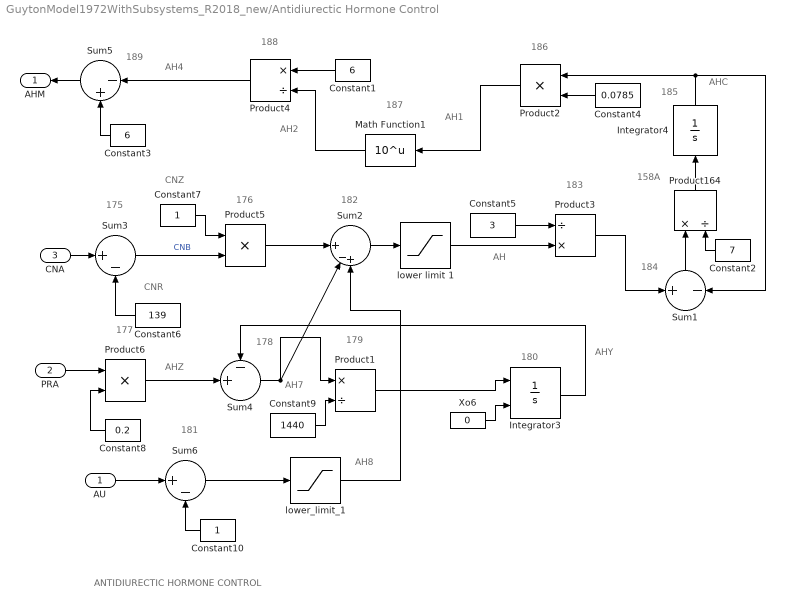
== system GuytonModel1972WithSubsystems_R2018_new/Antidiurectic Hormone Control ==
  note: AH4
  note: 175
  note: AH2
  note: 176
  note: AH1
  note: 184
  note: 182
  note: 183
  note: 180
  note: 158A
  note: 185
  note: 179
  note: 178
  note: 187
  note: 177
  note: 188
  note: ANTIDIURECTIC HORMONE CONTROL
  note: 186
  note: 189
  note: AHY
  note: CNZ
  note: CNR
  note: 181
  note: AH8
  note: AHC
  note: AH
  note: AHZ
  note: AH7
  AU : Inport
  PRA : Inport  Port=2
  CNA : Inport  Port=3
  Constant1 : Constant  Value=6
  Constant10 : Constant
  Constant2 : Constant  Value=7
  Constant3 : Constant  Value=6
  Constant4 : Constant  Value=0.0785
  Constant5 : Constant  Value=3
  Constant6 : Constant  Value=139
  Constant7 : Constant
  Constant8 : Constant  Value=0.2
  Constant9 : Constant  Value=1440
  Integrator3 : Integrator  InitialConditionSource=external
  Integrator4 : Integrator  InitialCondition=1
  Math Function1 : Math  Operator=10^u  SaturateOnIntegerOverflow=on
  Product1 : Product  Inputs=*/  SaturateOnIntegerOverflow=on  RndMeth=Zero  InputSameDT=on  OutDataTypeStr=Inherit: Same as first input
  Product164 : Product  Inputs=*/  SaturateOnIntegerOverflow=on  RndMeth=Zero  InputSameDT=on  OutDataTypeStr=Inherit: Same as first input
  Product2 : Product  SaturateOnIntegerOverflow=on  RndMeth=Zero  InputSameDT=on  OutDataTypeStr=Inherit: Same as first input
  Product3 : Product  Inputs=/*  SaturateOnIntegerOverflow=on  RndMeth=Zero  InputSameDT=on  OutDataTypeStr=Inherit: Same as first input
  Product4 : Product  Inputs=*/  SaturateOnIntegerOverflow=on  RndMeth=Zero  InputSameDT=on  OutDataTypeStr=Inherit: Same as first input
  Product5 : Product  SaturateOnIntegerOverflow=on  RndMeth=Zero  InputSameDT=on  OutDataTypeStr=Inherit: Same as first input
  Product6 : Product  SaturateOnIntegerOverflow=on  RndMeth=Zero  InputSameDT=on  OutDataTypeStr=Inherit: Same as first input
  Sum1 : Sum  Inputs=+|-  SaturateOnIntegerOverflow=on  InputSameDT=on  OutDataTypeStr=Inherit: Same as first input
  Sum2 : Sum  Inputs=|||+|-+  SaturateOnIntegerOverflow=on  InputSameDT=on  OutDataTypeStr=Inherit: Same as first input
  Sum3 : Sum  Inputs=|+-  SaturateOnIntegerOverflow=on  InputSameDT=on  OutDataTypeStr=Inherit: Same as first input
  Sum4 : Sum  Inputs=-+|  SaturateOnIntegerOverflow=on  InputSameDT=on  OutDataTypeStr=Inherit: Same as first input
  Sum5 : Sum  Inputs=|-+  SaturateOnIntegerOverflow=on  InputSameDT=on  OutDataTypeStr=Inherit: Same as first input
  Sum6 : Sum  Inputs=|+-  SaturateOnIntegerOverflow=on  InputSameDT=on  OutDataTypeStr=Inherit: Same as first input
  Xo6 : Constant  Value=0  VectorParams1D=off
  lower limit 1 : Saturate  UpperLimit=inf  LowerLimit=0  LinearizeAsGain=off
  lower_limit_1 : Saturate  UpperLimit=inf  LowerLimit=0  LinearizeAsGain=off
  AHM : Outport
  wires:
  Sum3/1 -> Product5/2  "CNB"
  Sum1/1 -> Product164/1
  Product164/1 -> Integrator4/1
  Constant1/1 -> Product4/1
  Product1/1 -> Integrator3/1
  Constant8/1 -> Product6/2
  Constant2/1 -> Product164/2
  Sum6/1 -> lower_limit_1/1
  Constant7/1 -> Product5/1
  Constant9/1 -> Product1/2
  Math Function1/1 -> Product4/2
  Product2/1 -> Math Function1/1
  Sum4/1 -> Product1/1, Sum2/2
  Xo6/1 -> Integrator3/2
  Constant4/1 -> Product2/2
  lower limit 1/1 -> Product3/2
  Integrator4/1 -> Product2/1, Sum1/2
  Sum2/1 -> lower limit 1/1
  Constant6/1 -> Sum3/2
  lower_limit_1/1 -> Sum2/3
  Integrator3/1 -> Sum4/1
  Product6/1 -> Sum4/2
  Constant3/1 -> Sum5/2
  Constant10/1 -> Sum6/2
  Constant5/1 -> Product3/1
  Product4/1 -> Sum5/1
  Product3/1 -> Sum1/1
  Product5/1 -> Sum2/1
  AU/1 -> Sum6/1
  PRA/1 -> Product6/1
  CNA/1 -> Sum3/1
  Sum5/1 -> AHM/1
